simulink model "stupidstupidnew20190311_pitch"  (R2017b)
settings: Solver=VariableStepAuto  StartTime=0.0  StopTime=100  RelTol=1e-7
libraries: simulink x4, etargetslib x1, dspnetwork x1, X_Plane_Communication_Library x1
settings Model: Creator=E6320  LastModifiedBy=DELL
settings SolverCC: AlgebraicLoopSolver=LineSearch
settings DataIOCC: SaveOutput=off  SignalLogging=off  DSMLogging=off  SaveTime=off
settings CodeAppCC: StateflowObjectComments=on

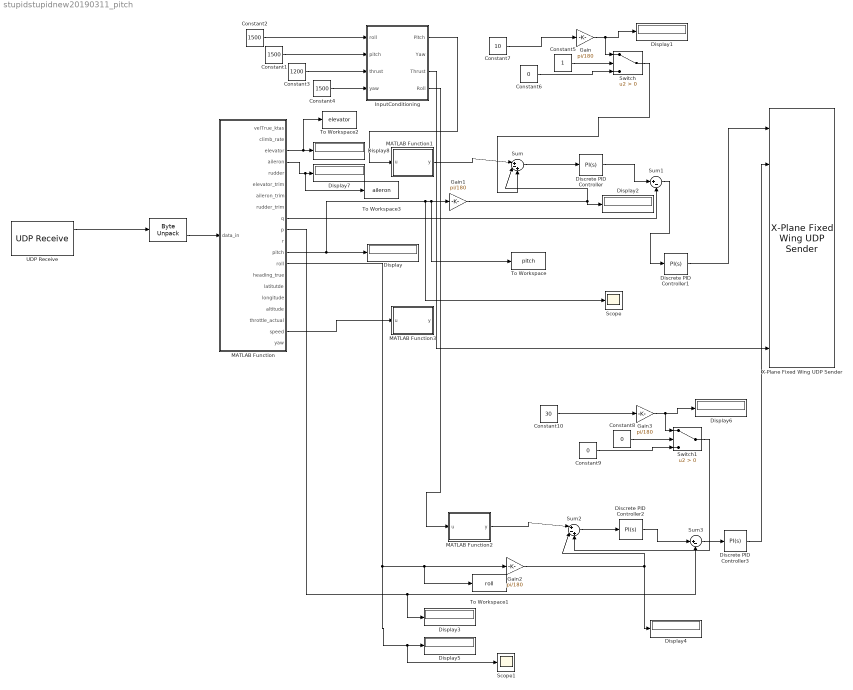
== system stupidstupidnew20190311_pitch ==
  "     " : etargetslib/Byte Unpack  dimensions={5,[9,21]}  datatypes={'uint8','single'}  byteAlign=1
  Constant1 : Constant  Value=1500
  Constant10 : Constant  Value=30
  Constant2 : Constant  Value=1500
  Constant3 : Constant  Value=1200
  Constant4 : Constant  Value=1500
  Constant5 : Constant
  Constant6 : Constant  Value=0
  Constant7 : Constant  Value=10
  Constant8 : Constant  Value=0
  Constant9 : Constant  Value=0
  Discrete PID Controller : simulink/Continuous/PID Controller  Controller=PI  TimeDomain=Continuous-time  SampleTime=-1  IntegratorMethod=Forward Euler  FilterMethod=Forward Euler  Form=Parallel  UseFilter=on  ControllerParametersSource=internal  P=1.8545410952272  I=2.0387841436751  D=0  N=100  InitialConditionSource=internal  InitialConditionForIntegrator=0  InitialConditionForFilter=0  ExternalReset=none  LimitOutput=off  UpperSaturationLimit=inf  LowerSaturationLimit=-inf  LinearizeAsGain=off  AntiWindupMode=none  Kb=1  TrackingMode=off  Kt=1  PParamMin=[]  PParamMax=[]  IParamMin=[]  IParamMax=[]  DParamMin=[]  DParamMax=[]  NParamMin=[]  NParamMax=[]  KbParamMin=[]  KbParamMax=[]  KtParamMin=[]  KtParamMax=[]  POutMin=[]  POutMax=[]  IOutMin=[]  IOutMax=[]  DOutMin=[]  DOutMax=[]  NOutMin=[]  NOutMax=[]  KbOutMin=[]  KbOutMax=[]  KtOutMin=[]  KtOutMax=[]  IntegratorOutMin=[]  IntegratorOutMax=[]  FilterOutMin=[]  FilterOutMax=[]  SumOutMin=[]  SumOutMax=[]  SumI1OutMin=[]  SumI1OutMax=[]  SumI2OutMin=[]  SumI2OutMax=[]  SumI3OutMin=[]  SumI3OutMax=[]  SumDOutMin=[]  SumDOutMax=[]  SaturationOutMin=[]  SaturationOutMax=[]  IntegratorContinuousStateAttributes=''  IntegratorStateMustResolveToSignalObject=off  IntegratorRTWStateStorageClass=Auto  FilterContinuousStateAttributes=''  FilterStateMustResolveToSignalObject=off  FilterRTWStateStorageClass=Auto  DifferentiatorICPrevScaledInput=0  DifferentiatorOutMin=[]  DifferentiatorOutMax=[]  InitialConditionSetting=State (most efficient)  FilterDiffOutCoefMin=[]  FilterDiffOutCoefMax=[]  SumDenOutMin=[]  SumDenOutMax=[]  SumNumOutMin=[]  SumNumOutMax=[]  ReciprocalOutMin=[]  ReciprocalOutMax=[]  DivideOutMin=[]  DivideOutMax=[]  TunerSelectOption=Transfer Function Based (PID Tuner App)
  Discrete PID Controller1 : simulink/Continuous/PID Controller  Controller=PI  TimeDomain=Continuous-time  SampleTime=-1  IntegratorMethod=Forward Euler  FilterMethod=Forward Euler  Form=Parallel  UseFilter=on  ControllerParametersSource=internal  P=0.9259440556509936  I=0.746476159593003  D=0  N=100  InitialConditionSource=internal  InitialConditionForIntegrator=0  InitialConditionForFilter=0  ExternalReset=none  LimitOutput=off  UpperSaturationLimit=inf  LowerSaturationLimit=-inf  LinearizeAsGain=off  AntiWindupMode=none  Kb=1  TrackingMode=off  Kt=1  PParamMin=[]  PParamMax=[]  IParamMin=[]  IParamMax=[]  DParamMin=[]  DParamMax=[]  NParamMin=[]  NParamMax=[]  KbParamMin=[]  KbParamMax=[]  KtParamMin=[]  KtParamMax=[]  POutMin=[]  POutMax=[]  IOutMin=[]  IOutMax=[]  DOutMin=[]  DOutMax=[]  NOutMin=[]  NOutMax=[]  KbOutMin=[]  KbOutMax=[]  KtOutMin=[]  KtOutMax=[]  IntegratorOutMin=[]  IntegratorOutMax=[]  FilterOutMin=[]  FilterOutMax=[]  SumOutMin=[]  SumOutMax=[]  SumI1OutMin=[]  SumI1OutMax=[]  SumI2OutMin=[]  SumI2OutMax=[]  SumI3OutMin=[]  SumI3OutMax=[]  SumDOutMin=[]  SumDOutMax=[]  SaturationOutMin=[]  SaturationOutMax=[]  IntegratorContinuousStateAttributes=''  IntegratorStateMustResolveToSignalObject=off  IntegratorRTWStateStorageClass=Auto  FilterContinuousStateAttributes=''  FilterStateMustResolveToSignalObject=off  FilterRTWStateStorageClass=Auto  DifferentiatorICPrevScaledInput=0  DifferentiatorOutMin=[]  DifferentiatorOutMax=[]  InitialConditionSetting=State (most efficient)  FilterDiffOutCoefMin=[]  FilterDiffOutCoefMax=[]  SumDenOutMin=[]  SumDenOutMax=[]  SumNumOutMin=[]  SumNumOutMax=[]  ReciprocalOutMin=[]  ReciprocalOutMax=[]  DivideOutMin=[]  DivideOutMax=[]  TunerSelectOption=Transfer Function Based (PID Tuner App)
  Discrete PID Controller2 : simulink/Continuous/PID Controller  Controller=PI  TimeDomain=Continuous-time  SampleTime=-1  IntegratorMethod=Forward Euler  FilterMethod=Forward Euler  Form=Parallel  UseFilter=on  ControllerParametersSource=internal  P=1.10009301262288  I=0.0135349169634299  D=0  N=100  InitialConditionSource=internal  InitialConditionForIntegrator=0  InitialConditionForFilter=0  ExternalReset=none  LimitOutput=off  UpperSaturationLimit=inf  LowerSaturationLimit=-inf  LinearizeAsGain=off  AntiWindupMode=none  Kb=1  TrackingMode=off  Kt=1  PParamMin=[]  PParamMax=[]  IParamMin=[]  IParamMax=[]  DParamMin=[]  DParamMax=[]  NParamMin=[]  NParamMax=[]  KbParamMin=[]  KbParamMax=[]  KtParamMin=[]  KtParamMax=[]  POutMin=[]  POutMax=[]  IOutMin=[]  IOutMax=[]  DOutMin=[]  DOutMax=[]  NOutMin=[]  NOutMax=[]  KbOutMin=[]  KbOutMax=[]  KtOutMin=[]  KtOutMax=[]  IntegratorOutMin=[]  IntegratorOutMax=[]  FilterOutMin=[]  FilterOutMax=[]  SumOutMin=[]  SumOutMax=[]  SumI1OutMin=[]  SumI1OutMax=[]  SumI2OutMin=[]  SumI2OutMax=[]  SumI3OutMin=[]  SumI3OutMax=[]  SumDOutMin=[]  SumDOutMax=[]  SaturationOutMin=[]  SaturationOutMax=[]  IntegratorContinuousStateAttributes=''  IntegratorStateMustResolveToSignalObject=off  IntegratorRTWStateStorageClass=Auto  FilterContinuousStateAttributes=''  FilterStateMustResolveToSignalObject=off  FilterRTWStateStorageClass=Auto  DifferentiatorICPrevScaledInput=0  DifferentiatorOutMin=[]  DifferentiatorOutMax=[]  InitialConditionSetting=State (most efficient)  FilterDiffOutCoefMin=[]  FilterDiffOutCoefMax=[]  SumDenOutMin=[]  SumDenOutMax=[]  SumNumOutMin=[]  SumNumOutMax=[]  ReciprocalOutMin=[]  ReciprocalOutMax=[]  DivideOutMin=[]  DivideOutMax=[]  TunerSelectOption=Transfer Function Based (PID Tuner App)
  Discrete PID Controller3 : simulink/Continuous/PID Controller  Controller=PI  TimeDomain=Continuous-time  SampleTime=-1  IntegratorMethod=Forward Euler  FilterMethod=Forward Euler  Form=Parallel  UseFilter=on  ControllerParametersSource=internal  P=0.0549143230570902  I=1.1637891162682  D=0  N=100  InitialConditionSource=internal  InitialConditionForIntegrator=0  InitialConditionForFilter=0  ExternalReset=none  LimitOutput=off  UpperSaturationLimit=inf  LowerSaturationLimit=-inf  LinearizeAsGain=off  AntiWindupMode=none  Kb=1  TrackingMode=off  Kt=1  PParamMin=[]  PParamMax=[]  IParamMin=[]  IParamMax=[]  DParamMin=[]  DParamMax=[]  NParamMin=[]  NParamMax=[]  KbParamMin=[]  KbParamMax=[]  KtParamMin=[]  KtParamMax=[]  POutMin=[]  POutMax=[]  IOutMin=[]  IOutMax=[]  DOutMin=[]  DOutMax=[]  NOutMin=[]  NOutMax=[]  KbOutMin=[]  KbOutMax=[]  KtOutMin=[]  KtOutMax=[]  IntegratorOutMin=[]  IntegratorOutMax=[]  FilterOutMin=[]  FilterOutMax=[]  SumOutMin=[]  SumOutMax=[]  SumI1OutMin=[]  SumI1OutMax=[]  SumI2OutMin=[]  SumI2OutMax=[]  SumI3OutMin=[]  SumI3OutMax=[]  SumDOutMin=[]  SumDOutMax=[]  SaturationOutMin=[]  SaturationOutMax=[]  IntegratorContinuousStateAttributes=''  IntegratorStateMustResolveToSignalObject=off  IntegratorRTWStateStorageClass=Auto  FilterContinuousStateAttributes=''  FilterStateMustResolveToSignalObject=off  FilterRTWStateStorageClass=Auto  DifferentiatorICPrevScaledInput=0  DifferentiatorOutMin=[]  DifferentiatorOutMax=[]  InitialConditionSetting=State (most efficient)  FilterDiffOutCoefMin=[]  FilterDiffOutCoefMax=[]  SumDenOutMin=[]  SumDenOutMax=[]  SumNumOutMin=[]  SumNumOutMax=[]  ReciprocalOutMin=[]  ReciprocalOutMax=[]  DivideOutMin=[]  DivideOutMax=[]  TunerSelectOption=Transfer Function Based (PID Tuner App)
  Display{,1..8} (9 alike) : Display
  Gain{,1..3} (4 alike) : Gain  Gain=pi/180
  InputConditioning : Subsystem
  MATLAB Function : MATLAB Function  TreatAsAtomicUnit=on
  MATLAB Function1 : MATLAB Function  TreatAsAtomicUnit=on
  MATLAB Function2 : MATLAB Function  TreatAsAtomicUnit=on
  MATLAB Function3 : MATLAB Function  TreatAsAtomicUnit=on
  Scope : Scope
  Scope1 : Scope
  Sum : Sum  Inputs=|+-+
  Sum1 : Sum  Inputs=|+-
  Sum2 : Sum  Inputs=|+-+
  Sum3 : Sum  Inputs=|+-
  Switch : Switch  Criteria=u2 > Threshold
  Switch1 : Switch  Criteria=u2 > Threshold
  To Workspace : ToWorkspace  VariableName=pitch  SaveFormat=Timeseries  SampleTime=-1
  To Workspace1 : ToWorkspace  VariableName=roll  SaveFormat=Timeseries  SampleTime=-1
  To Workspace2 : ToWorkspace  VariableName=elevator  SaveFormat=Timeseries  SampleTime=-1
  To Workspace3 : ToWorkspace  VariableName=aileron  SaveFormat=Timeseries  SampleTime=-1
  UDP Receive : dspnetwork/UDP Receive  localURL='0.0.0.0'  localPort=49004  remoteURL='127.0.0.1'  remotePort=-1  recvBufferSize=8192  dims=761  signalDatatype=uint8  isVarSize=off  showBlockingTime=on  blockingTime=10  sampletime=0.02  blockPlatform=HOST
      settings: SourceProductName=DSP System Toolbox  SourceProductBaseCode=DS
  X-Plane Fixed Wing UDP Sender : X_Plane_Communication_Library/Fixed Wing/X-Plane Fixed Wing UDP Sender  ip_adress='127.0.0.1'  port_number=49000
  wires:
  UDP Receive/1 -> "     "/1
  "     "/2 -> MATLAB Function/1(data_in)
  Constant3/1 -> InputConditioning/3(thrust)
  Constant4/1 -> InputConditioning/4(yaw)
  Constant2/1 -> InputConditioning/1(roll)
  Constant1/1 -> InputConditioning/2(pitch)
  MATLAB Function1/1(y) -> Sum/1
  Sum/1 -> Discrete PID Controller/1
  MATLAB Function/12(pitch) -> Scope/1, To Workspace/1, Gain1/1, Display/1
  Gain/1 -> Switch/1, Display1/1
  Constant7/1 -> Gain/1
  Gain1/1 -> Display2/1, Sum/2
  Constant6/1 -> Switch/3
  Constant5/1 -> Switch/2
  Switch/1 -> Sum/3
  InputConditioning/1(Pitch) -> MATLAB Function1/1(u)
  Discrete PID Controller/1 -> Sum1/1
  Sum1/1 -> Discrete PID Controller1/1
  Discrete PID Controller1/1 -> X-Plane Fixed Wing UDP Sender/1
  MATLAB Function/9(q) -> Sum1/2
  MATLAB Function/19(speed) -> MATLAB Function3/1(u)
  Sum2/1 -> Discrete PID Controller2/1
  InputConditioning/4(Roll) -> MATLAB Function2/1(u)
  Sum3/1 -> Discrete PID Controller3/1
  MATLAB Function/10(p) -> Display3/1, Sum3/2
  Gain2/1 -> Display4/1, Sum2/2
  MATLAB Function2/1(y) -> Sum2/1
  Discrete PID Controller3/1 -> X-Plane Fixed Wing UDP Sender/2
  MATLAB Function/13(roll) -> Scope1/1, Display5/1, To Workspace1/1, Gain2/1
  Switch1/1 -> Sum2/3
  Discrete PID Controller2/1 -> Sum3/1
  Gain3/1 -> Switch1/1, Display6/1
  Constant9/1 -> Switch1/3
  Constant8/1 -> Switch1/2
  Constant10/1 -> Gain3/1
  InputConditioning/3(Thrust) -> X-Plane Fixed Wing UDP Sender/7
  MATLAB Function/4(aileron) -> To Workspace3/1, Display7/1
  MATLAB Function/3(elevator) -> To Workspace2/1, Display8/1

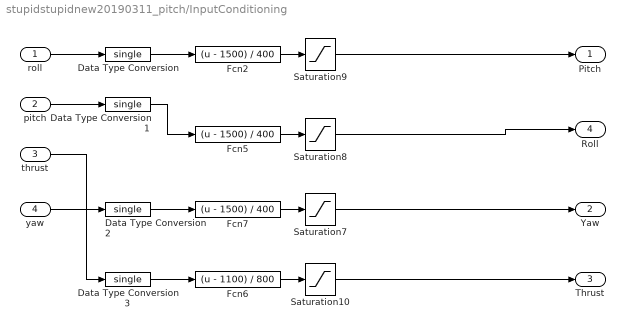
== system stupidstupidnew20190311_pitch/InputConditioning ==
  roll : Inport
  pitch : Inport  Port=2
  thrust : Inport  Port=3
  yaw : Inport  Port=4
  Data Type Conversion{,1..3} (4 alike) : DataTypeConversion  OutDataTypeStr=single
  Fcn2 : Fcn  Expr=(u - 1500) / 400
  Fcn5 : Fcn  Expr=(u - 1500) / 400
  Fcn6 : Fcn  Expr=(u - 1100) / 800
  Fcn7 : Fcn  Expr=(u - 1500) / 400
  Saturation10 : Saturate  UpperLimit=1  LowerLimit=0
  Saturation7 : Saturate  UpperLimit=1  LowerLimit=-1
  Saturation8 : Saturate  UpperLimit=1  LowerLimit=-1
  Saturation9 : Saturate  UpperLimit=1  LowerLimit=-1
  Pitch : Outport
  Yaw : Outport  Port=2
  Thrust : Outport  Port=3
  Roll : Outport  Port=4
  wires:
  Saturation10/1 -> Thrust/1
  Saturation9/1 -> Pitch/1
  Fcn6/1 -> Saturation10/1
  thrust/1 -> Data Type Conversion3/1
  Fcn2/1 -> Saturation9/1
  Fcn5/1 -> Saturation8/1
  Fcn7/1 -> Saturation7/1
  yaw/1 -> Data Type Conversion2/1
  pitch/1 -> Data Type Conversion1/1
  roll/1 -> Data Type Conversion/1
  Data Type Conversion/1 -> Fcn2/1
  Data Type Conversion1/1 -> Fcn5/1
  Data Type Conversion2/1 -> Fcn7/1
  Data Type Conversion3/1 -> Fcn6/1
  Saturation8/1 -> Roll/1
  Saturation7/1 -> Yaw/1

== matlab function stupidstupidnew20190311_pitch/MATLAB Function1 ==
  data: u input; y output
function y = fcn(u)

y = round(u*100)/100;

== matlab function stupidstupidnew20190311_pitch/MATLAB Function ==
  data: data_in input; velTrue_ktas output; climb_rate output; elevator output; aileron output; rudder output; elevator_trim output; aileron_trim output; rudder_trim output; q output; p output; r output; pitch output; roll output; heading_true output; latitutde output; longitude output; altitude output; throttle_actual output; speed output; yaw output
function [velTrue_ktas, climb_rate,elevator, aileron, rudder, elevator_trim, aileron_trim, rudder_trim, q,p,r, pitch, roll, heading_true, latitutde, longitude, altitude, throttle_actual,speed,yaw]   = fcn(data_in)
% This block supports the Embedded MATLAB subset.
% See the help menu for details. 


velTrue_ktas = data_in(4,1);

climb_rate = data_in(4,2);

elevator = data_in(2,3);
aileron = data_in(3,3);
rudder= data_in(4,3);


elevator_trim= data_in(2,4);
aileron_trim= data_in(3,4);
rudder_trim= data_in(4,4);

q= data_in(2,5);
p= data_in(3,5);
r= data_in(4,5);
yaw = data_in(5,5);

pitch= data_in(2,6);
roll= data_in(3,6);
heading_true= data_in(4,6);

latitutde= data_in(2,7);
longitude= data_in(3,7);

altitude= data_in(4,7);
throttle_actual = data_in(2,8);
speed = data_in(2,2);

== matlab function stupidstupidnew20190311_pitch/MATLAB Function2 ==
  data: u input; y output
function y = fcn(u)

y = round(u*100)/100;

== matlab function stupidstupidnew20190311_pitch/MATLAB Function3 ==
  data: u input; y output
function y = fcn(u)
if(u<=0.0308)
y = 0.15;
else
    y=0
end
